simulink model "model_p1"  (R2020b)
settings: Solver=VariableStepAuto  StartTime=0.0  StopTime=10.0  RelTol=1e-3
model workspace (MAT data in the model file):
  K1 = 50
  M1 = 100
  b = 50
settings Model: OrderedModelArguments=off  Creator=ADMIN  LastModifiedBy=ADMIN

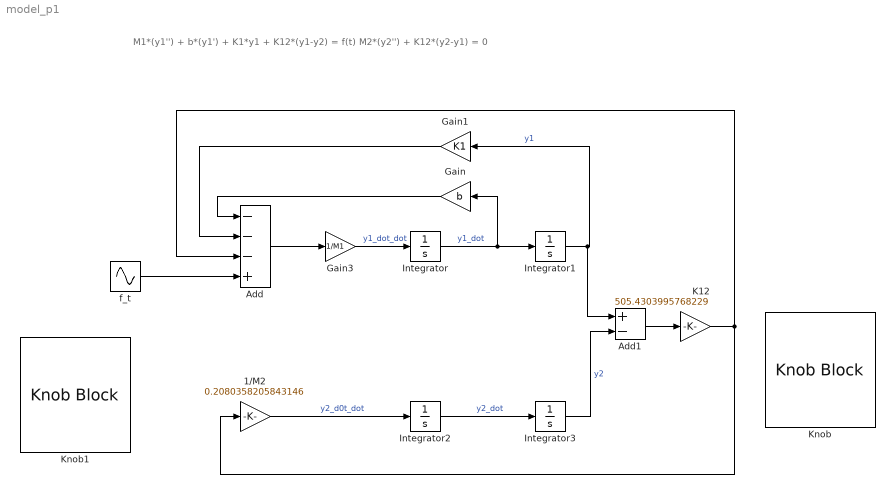
== system model_p1 ==
  note: M1*(y1'') + b*(y1') + K1*y1 + K12*(y1-y2) = f(t)
      | M2*(y2'') + K12*(y2-y1) = 0
  1/M2 : Gain  Gain=0.2080358205843146
  Add : Sum  Inputs=---+
  Add1 : Sum  Inputs=+-
  Gain : Gain  Gain=b
  Gain1 : Gain  Gain=K1
  Gain3 : Gain  Gain=1/M1
  Integrator{,1..3} (4 alike) : Integrator
  K12 : Gain  Gain=505.4303995768229
  Knob : KnobBlock  ScaleMax=1000
  Knob1 : KnobBlock  ScaleMin=0.1  ScaleMax=1
  f_t : Sin  Amplitude=2  Frequency=10  SampleTime=0.01
  wires:
  Gain3/1 -> Integrator/1  "y1_dot_dot"
  Integrator/1 -> Gain/1, Integrator1/1  "y1_dot"
  Integrator1/1 -> Gain1/1, Add1/1  "y1"
  1/M2/1 -> Integrator2/1  "y2_d0t_dot"
  Integrator2/1 -> Integrator3/1  "y2_dot"
  Integrator3/1 -> Add1/2  "y2"
  f_t/1 -> Add/4
  Gain/1 -> Add/1
  Gain1/1 -> Add/2
  Add1/1 -> K12/1
  K12/1 -> 1/M2/1, Add/3
  Add/1 -> Gain3/1
